simulink subsystem "PvtSubSys_HMI"  (R2020b)
settings: Solver=VariableStepAuto  StartTime=0.0  StopTime=10.0  RelTol=1e-3
undefined symbols (not defined in the file): P_HMI_LDW_LKAWarnTime, P_HMI_ObjectTypeFilter, P_HMI_WarnFormLDWReq
libraries: simulink x212, TrueDurationTime x6
(part 2 of 8)

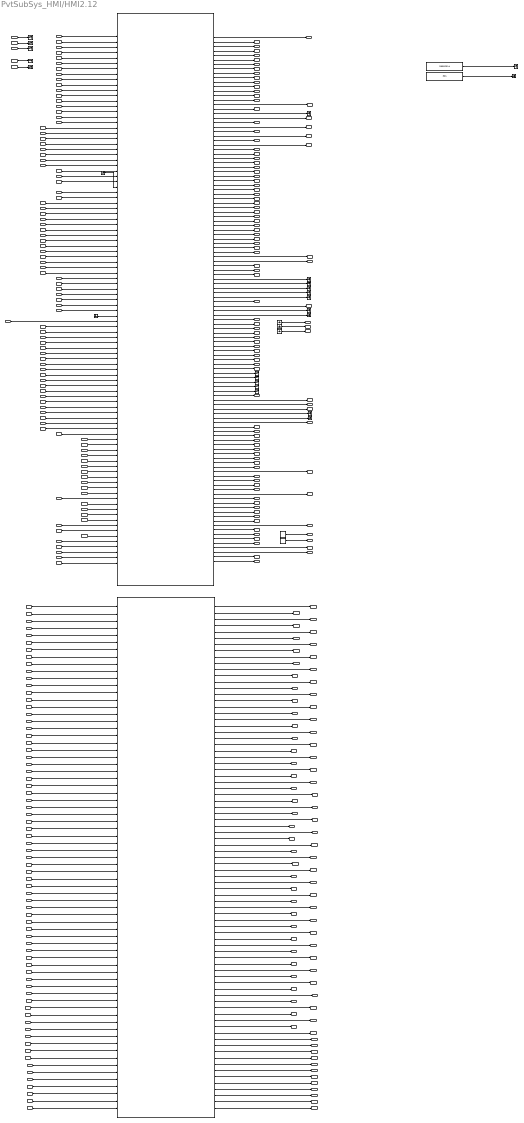
== system PvtSubSys_HMI/HMI2.12 ==
  note: 新加
  note: 与下 名字不一致
  note: 输出信号：拉出皆为输入与输出名字相同导致
      | 绿色：ACC_FD1
      | 黄色：ACC_FD2
  note: notuse
  ACCSts : Inport
  ACC_SpdSetValue : Inport  Port=2
  ACC_TimeGapSet : Inport  Port=3
  ACC_DrvOffReq : Inport  Port=4
  vSetBelowMin : Inport  Port=5
  HWAAccControlSts : Inport  Port=6
  TJASts : Inport  Port=7
  HWASts : Inport  Port=8
  HWAActive : Inport  Port=9
  ACC_HazActv : Inport  Port=10
  ACC_ModeDisp : Inport  Port=11
  ACC_ParkShiftReq : Inport  Port=12
  TJA_ModeDisp : Inport  Port=13
  HWA_ModeDisp : Inport  Port=14
  HWASlowRetreat_b : Inport  Port=15
  CruiseChauffeur_ModeDisp : Inport  Port=16
  ACCTextDisp : Inport  Port=17
  TJATextDisp : Inport  Port=18
  CCTextDisp : Inport  Port=19
  HWATextDisp : Inport  Port=20
  LCKSts : Inport  Port=21
  HandsOffWarningLevel : Inport  Port=22
  LDWState : Inport  Port=23
  LKAState : Inport  Port=24
  LKAWarning : Inport  Port=25
  ELKSts : Inport  Port=26
  LCKIESts : Inport  Port=27
  ACC_ISLResp : Inport  Port=28
  ISL_InterSysInfoDisp : Inport  Port=29
  ISLActive : Inport  Port=30
  ALC_Resp : Inport  Port=31
  HWA_SnvtySet_Resp : Inport  Port=32
  HWA_Resp : Inport  Port=33
  ICA_HandsOffSwtResp : Inport  Port=34
  TJA_ACC_SelSts : Inport  Port=35
  HWA_LaneChangeReq : Inport  Port=36
  HWA_Warning : Inport  Port=37
  HandsoffDetd : Inport  Port=38
  LSS_WarnFormSwtResp : Inport  Port=39
  DriverInloop_Monitor : Inport  Port=40
  ACC_SOS_Req : Inport  Port=41
  LaneAvailability : Inport  Port=42
  TJA_FollowSts : Inport  Port=43
  ESSSts : Inport  Port=44
  AESSts : Inport  Port=45
  HWA_TurnLightReq : Inport  Port=46
  ACC_DrvrOffDisp : Inport  Port=47
  LSSSwtReq : Inport  Port=48
  ESS_PedSwtReq : Inport  Port=49
  ESS_VehSwtReq : Inport  Port=50
  AESSwtReq : Inport  Port=51
  IFC_SnvtySet : Inport  Port=52
  ADAS_Posn_CurLane : Inport  Port=53
  NavSpdLimValue : Inport  Port=54
  NavSpdLimUnit_HUT : Inport  Port=55
  IFC_CalibrationSts : Inport  Port=56
  Camera_BlockageSts : Inport  Port=57
  ACC_Decel_Req : Inport  Port=58
  IDP0 : Inport  Port=59
  dxP0 : Inport  Port=60
  vxRelP0 : Inport  Port=61
  ACCTgtObjVy : Inport  Port=62
  axAbsGroundP0 : Inport  Port=63
  targetExistP0 : Inport  Port=64
  fu_typeP0 : Inport  Port=65
  ObjMovingStateP0 : Inport  Port=66
  Object_Orientation : Inport  Port=67
  ObjTypeP0 : Inport  Port=68
  ObjDYP0 : Inport  Port=69
  ACCTgtObjObstcl : Inport  Port=70
  ACCTgtObjAy : Inport  Port=71
  ACCTgtObjCntAlive : Inport  Port=72
  ACCTgtObjExist : Inport  Port=73
  P0HeadingAngle : Inport  Port=74
  <IDP1> : Inport  Port=75
  dxP1 : Inport  Port=76
  targetExistP1 : Inport  Port=77
  fu_typeP1 : Inport  Port=78
  ObjTypeP1 : Inport  Port=79
  ObjDYP1 : Inport  Port=80
  P1HeadingAngle : Inport  Port=81
  IDP2 : Inport  Port=82
  dxP2 : Inport  Port=83
  targetExistP2 : Inport  Port=84
  fu_typeP2 : Inport  Port=85
  ObjTypeP2 : Inport  Port=86
  ObjDYP2 : Inport  Port=87
  P2HeadingAngle : Inport  Port=88
  IDP3 : Inport  Port=89
  dxP3 : Inport  Port=90
  targetExistP3 : Inport  Port=91
  fu_typeP3 : Inport  Port=92
  ObjTypeP3 : Inport  Port=93
  ObjDYP3 : Inport  Port=94
  P3HeadingAngle : Inport  Port=95
  dyP4 : Inport  Port=96
  dxP4 : Inport  Port=97
  ObjTypeP4 : Inport  Port=98
  targetExistP4 : Inport  Port=99
  dyP5 : Inport  Port=100
  dxP5 : Inport  Port=101
  ObjTypeP5 : Inport  Port=102
  targetExistP5 : Inport  Port=103
  "L1blsLineExist " : Inport  Port=104
  L1dC0V : Inport  Port=105
  L1dC1V : Inport  Port=106
  L1dC2V : Inport  Port=107
  L1dC3V : Inport  Port=108
  L1enLineType : Inport  Port=109
  L1dDisStart : Inport  Port=110
  L1dDisFront : Inport  Port=111
  "R1blsLineExist " : Inport  Port=112
  R1dC0V : Inport  Port=113
  R1dC1V : Inport  Port=114
  R1dC2V : Inport  Port=115
  R1dC3V : Inport  Port=116
  R1enLineType : Inport  Port=117
  R1dDisStart : Inport  Port=118
  R1dDisFront : Inport  Port=119
  L2dC0V : Inport  Port=120
  L2dC1V : Inport  Port=121
  L2dC2V : Inport  Port=122
  L2dC3V : Inport  Port=123
  L2enLineType : Inport  Port=124
  L2dDisStart : Inport  Port=125
  L2dDisFront : Inport  Port=126
  L2LineExist : Inport  Port=127
  R2dC0V : Inport  Port=128
  R2dC1V : Inport  Port=129
  R2dC2V : Inport  Port=130
  R2dC3V : Inport  Port=131
  R2enLineType : Inport  Port=132
  R2dDisStart : Inport  Port=133
  R2dDisFront : Inport  Port=134
  R2LineExist : Inport  Port=135
  F_LBblsLineExist : Inport  Port=136
  F_LBdC0V : Inport  Port=137
  F_LBdC1V : Inport  Port=138
  F_LBdC2V : Inport  Port=139
  F_LBdC3V : Inport  Port=140
  F_LBenLineType : Inport  Port=141
  E1dDisStart : Inport  Port=142
  E1dDisFront : Inport  Port=143
  F_RBblsLineExist : Inport  Port=144
  F_RBdC0V : Inport  Port=145
  F_RBdC1V : Inport  Port=146
  F_RBdC2V : Inport  Port=147
  F_RBdC3V : Inport  Port=148
  F_RBenLineType : Inport  Port=149
  E2dDisFront : Inport  Port=150
  E2dDisStart : Inport  Port=151
  TunnelDistance : Inport  Port=152
  BridgeDistance : Inport  Port=153
  RampDistance : Inport  Port=154
  DrivingOnHighWay : Inport  Port=155
  RoadCurvatureFarDistance : Inport  Port=156
  RoadCurvature : Inport  Port=157
  RoadCurvatureFar : Inport  Port=158
  "Inter_AEB_TgtDecel_Req " : Inport  Port=159
  Inter_FCW_Warn : Inport  Port=160
  TSR_Sign_Long_Distance : Inport  Port=161
  DrvrState : Inport  Port=162
  MapDataValid : Inport  Port=163
  IFCHUTInterface : Inport  Port=164
  Long_ACCTakeoverReq : Inport  Port=165
  ACC_TgtObjBarDisp : Inport  Port=166
  ACC_LeTgtObjBarDisp : Inport  Port=167
  ACC_RiTgtObjBarDisp : Inport  Port=168
  LKASwtReq : Inport  Port=169
  LCKSwtReq : Inport  Port=170
  IntelligentCurveActive : Inport  Port=171
  standstill : Inport  Port=172
  Constant : Constant  Value=false
  Constant2 : Constant  Value=0  OutDataTypeStr=uint8
  Constant7 : Constant  Value=39092014  OutDataTypeStr=uint32
  Constant8 : Constant  Value=301  OutDataTypeStr=uint16
  Ground{3,10,12..14} (5 alike) : Ground
  HWA/ACC/TJA_Signal1 : Subsystem
  IFC_Signal1 : Subsystem
  TJASts1 : InportShadow  Port=7
  Terminator{1..3,5..6,9..22,24..26} (22 alike) : Terminator
  ACC_ModDisp : Outport
  TJA_ICA_ModDisp : Outport  Port=2
  HWA_ModDisp : Outport  Port=3
  ACC_InterSysInfoDisp : Outport  Port=4
  TJA_ICA_InterSysInfoDisp : Outport  Port=5
  HWA_InterSysInfoDisp : Outport  Port=6
  CruCha_ModDisp : Outport  Port=7
  CruChar_InterSysInfoDisp : Outport  Port=8
  ALCResp : Outport  Port=9
  HWAResp : Outport  Port=10
  ISL_Resp : Outport  Port=11
  ICA_HandsOffResp : Outport  Port=12
  HWAwarning : Outport  Port=13
  ACCTimeGapSet : Outport  Port=14
  ACCSpdSetValue : Outport  Port=15
  TJA_ACCSelSts : Outport  Port=16
  ACC_TakeOverReq : Outport  Port=17
  ACC_FctSts : Outport  Port=18
  ACC_EgoStatus : Outport  Port=19
  Longctrl_HazActv : Outport  Port=20
  ADAS_DriverInloop_Monitor : Outport  Port=21
  HWASnvtySetResp : Outport  Port=22
  HWA_Lane_ChangeReq : Outport  Port=23
  HWA_LaneChange : Outport  Port=24
  ACC_ObjDetecte : Outport  Port=25
  ACC_RlvTgtDetn : Outport  Port=26
  ACC_PotentialTgtDetn : Outport  Port=27
  ACC_PotentialTgtTyp : Outport  Port=28
  ACC_PotentialTgtDx : Outport  Port=29
  ACC_PotentialTgtDy : Outport  Port=30
  ACC_LeTargrtDection : Outport  Port=31
  ACC_LeTgtTyp : Outport  Port=32
  ACC_LeTgtDx : Outport  Port=33
  ACC_LeTgtDy : Outport  Port=34
  ACC_RiTargrtDetn : Outport  Port=35
  ACC_RiTgtTyp : Outport  Port=36
  ACC_RiTgtDx : Outport  Port=37
  ACC_RiTgtDy : Outport  Port=38
  ISLInterSysInfoDisp : Outport  Port=39
  Longctrl_DrvOFF_Req_DVR : Outport  Port=40
  Longctrl_ModSts_DVR : Outport  Port=41
  Longctrl_ParkShiftReq_DVR : Outport  Port=42
  ACC_RlvTgtTyp : Outport  Port=43
  ACC_RlvTgtDx : Outport  Port=44
  ACC_RlvTgtDy : Outport  Port=45
  Longctrl_HCUTrqReq_DVR : Outport  Port=46
  ALC_InterSysInfoDisp : Outport  Port=47
  Request_driveoff : Outport  Port=48
  Longctrl_VehHldReq_DVR : Outport  Port=49
  Longctrl_HCUTrqReqActive_DVR : Outport  Port=50
  IntelligentCurveAct : Outport  Port=51
  ACC_RlvTgtfusion : Outport  Port=52
  ACC_RlvTgtHeading : Outport  Port=53
  ACC_LeTgtfusion : Outport  Port=54
  ACC_LeTgtHeading : Outport  Port=55
  ACC_RiTgtfusion : Outport  Port=56
  ACC_RiTgtHeading : Outport  Port=57
  ACC_PotentialTgtfusion : Outport  Port=58
  ACC_PotentialTgtHeading : Outport  Port=59
  ACC_LeTgt_02_Dy : Outport  Port=60
  ACC_LeTgt_02_Dx : Outport  Port=61
  ACC_LeTgt_02_Typ : Outport  Port=62
  ACC_LeTargrt_02_Detn : Outport  Port=63
  ACC_RiTargrt_02_Detn : Outport  Port=64
  ACC_RiTgt_02_Dy : Outport  Port=65
  ACC_RiTgt_02_Dx : Outport  Port=66
  ACC_RiTgt_02_Typ : Outport  Port=67
  ACCTgtObjBarDisp : Outport  Port=68
  ACCLeTgtObjBarDisp : Outport  Port=69
  ACCRiTgtObjBarDisp : Outport  Port=70
  Longctrl_DrvOFF_Req : Outport  Port=71
  Longctrl_ModSts : Outport  Port=72
  Longctrl_ParkShiftReq : Outport  Port=73
  ActualTargetSpeed : Outport  Port=74
  Longctrl_VehHldReq : Outport  Port=75
  ACC_CRInterface : Outport  Port=76
  Longctrl_FuelCutOffPrevn : Outport  Port=77
  ACCTgtObjDx : Outport  Port=78
  ACCTgtObjDy : Outport  Port=79
  ACC_TgtObjObstcl : Outport  Port=80
  ACC_TgtObjExist : Outport  Port=81
  ACC_TgtObjVy : Outport  Port=82
  ACCTgtObjVx : Outport  Port=83
  ACCTgtObjAx : Outport  Port=84
  ACC_TgtObjAy : Outport  Port=85
  ACCTgtObjState : Outport  Port=86
  ACCTgtObjVideoCfmd : Outport  Port=87
  ACC_TgtObjCntAlive : Outport  Port=88
  Handsoff_Detd : Outport  Port=89
  DrvgOnHiWay : Outport  Port=90
  RoadCrvt : Outport  Port=91
  SpdLimitDst : Outport  Port=92
  RoadCrvtFar : Outport  Port=93
  RampDst : Outport  Port=94  OutDataTypeStr=uint16
  SpdLimit : Outport  Port=95
  CurveDst : Outport  Port=96
  NavSpdLimUnit : Outport  Port=97
  TunnelDst : Outport  Port=98  OutDataTypeStr=uint16
  Drvg_OnRiLane : Outport  Port=99
  BrdgDst : Outport  Port=100  OutDataTypeStr=uint16
  ACC_SOSReq : Outport  Port=101
  Map_DataValid : Outport  Port=102
  DrvrSts : Outport  Port=103
  ACCTgtObjID : Outport  Port=104
  LSSIntervention : Outport  Port=105
  LSSWarnFormResp : Outport  Port=106
  ELKResp : Outport  Port=107
  LCKResp : Outport  Port=108
  LKAResp : Outport  Port=109
  LDWResp : Outport  Port=110
  IntelligentEvaResp : Outport  Port=111
  LSSFuncSts : Outport  Port=112
  LSSErrSts : Outport  Port=113
  LSSResp : Outport  Port=114
  ELKMainState : Outport  Port=115
  LDW_LKAWarn : Outport  Port=116
  ESS_PedResp : Outport  Port=117
  ESS_VehResp : Outport  Port=118
  AESResp : Outport  Port=119
  IFC_LaneAvailability : Outport  Port=120
  LDW_LKA_Snvty : Outport  Port=121
  IFCCalibrationSts : Outport  Port=122
  IFC_HUTInterface : Outport  Port=123
  CameraBlockageSts : Outport  Port=124
  TJAFollowSts : Outport  Port=125
  IFC_LeLaneTyp : Outport  Port=126
  IFC_RiLaneTyp : Outport  Port=127
  IFC_NextLeLaneTyp : Outport  Port=128
  IFC_NextRiLaneTyp : Outport  Port=129
  IFC_LaneCurve : Outport  Port=130
  IFC_LeLane_dy : Outport  Port=131
  IFC_RiLane_dy : Outport  Port=132
  IFC_NextLeLane_dy : Outport  Port=133
  IFC_NextRiLane_dy : Outport  Port=134
  AESintervention : Outport  Port=135
  ESSintervention : Outport  Port=136
  ELKActSts : Outport  Port=137
  IntelligentEvaActSts : Outport  Port=138
  IFC_Handsoffwarn : Outport  Port=139
  AES_Sts : Outport  Port=140
  ESS_Sts : Outport  Port=141
  IFC_Line01_Dy : Outport  Port=142
  IFC_Line01_Curv : Outport  Port=143
  IFC_Line01_CurvChange : Outport  Port=144
  IFC_Line01_Type : Outport  Port=145
  IFC_Line02_Dy : Outport  Port=146
  IFC_Line02_Curv : Outport  Port=147
  IFC_Line02_CurvChange : Outport  Port=148
  IFC_Line02_Type : Outport  Port=149
  IFC_Line03_Dy : Outport  Port=150
  IFC_Line03_Curv : Outport  Port=151
  IFC_Line03_CurvChange : Outport  Port=152
  IFC_Line03_Type : Outport  Port=153
  IFC_Line04_Dy : Outport  Port=154
  IFC_Line04_Curv : Outport  Port=155
  IFC_Line04_CurvChange : Outport  Port=156
  IFC_Line04_Type : Outport  Port=157
  IFC_Roadedge01_Dy : Outport  Port=158
  IFC_Roadedge01_Curv : Outport  Port=159
  IFC_Roadedge01_CurvChange : Outport  Port=160
  IFC_Roadedge01_Type : Outport  Port=161
  IFC_Roadedge02_Dy : Outport  Port=162
  IFC_Roadedge02_Curv : Outport  Port=163
  IFC_Roadedge02_CurvChange : Outport  Port=164
  IFC_Roadedge02_Type : Outport  Port=165
  IFC_Line01_HeadingAngle : Outport  Port=166
  IFC_Line02_HeadingAngle : Outport  Port=167
  IFC_Line03_HeadingAngle : Outport  Port=168
  IFC_Line04_HeadingAngle : Outport  Port=169
  IFC_Roadedge01_HeadingAngle : Outport  Port=170
  IFC_Roadedge02_HeadingAngle : Outport  Port=171
  IFC_Line01_DxStart : Outport  Port=172
  IFC_Line01_DxEnd : Outport  Port=173
  IFC_Line02_DxStart : Outport  Port=174
  IFC_Line02_DxEnd : Outport  Port=175
  IFC_Line03_DxStart : Outport  Port=176
  IFC_Line03_DxEnd : Outport  Port=177
  IFC_Line04_DxStart : Outport  Port=178
  IFC_Line04_DxEnd : Outport  Port=179
  IFC_Roadedge01_DxStart : Outport  Port=180
  IFC_Roadedge01_DxEnd : Outport  Port=181
  IFC_Roadedge02_DxStart : Outport  Port=182
  IFC_Roadedge02_DxEnd : Outport  Port=183
  IFCVibrationWarning : Outport  Port=184
  AESErrSts : Outport  Port=185
  ESSErrSts : Outport  Port=186
  IDC_L2_EmgyLightReq : Outport  Port=187
  IDC_L2_TurnLightReq : Outport  Port=188
  IDC_L2_FWiperReq : Outport  Port=189
  wires:
  standstill/1 -> IFC_Signal1/71(standstill)
  Constant7/1 -> Terminator24/1  "HMI_SubModel_VERSION"
  Constant8/1 -> Terminator26/1  "HMI_SubModel_Number"
  ACC_DrvrOffDisp/1 -> HWA/ACC/TJA_Signal1/99(ACC_DrvrOffDisp)
  R2LineExist/1 -> IFC_Signal1/70(R2LineExist)
  L2LineExist/1 -> IFC_Signal1/69(L2LineExist)
  E2dDisFront/1 -> IFC_Signal1/68(E2dDisStart)
  E2dDisStart/1 -> IFC_Signal1/67(E2dDisFront)
  L2dDisStart/1 -> IFC_Signal1/61(L2dDisStart)
  R1dDisFront/1 -> IFC_Signal1/60(R1dDisFront)
  R1dDisStart/1 -> IFC_Signal1/59(R1dDisStart)
  L2dDisFront/1 -> IFC_Signal1/62(L2dDisFront)
  E1dDisFront/1 -> IFC_Signal1/66(E1dDisFront)
  R2dDisFront/1 -> IFC_Signal1/64(R2dDisFront)
  L1dDisFront/1 -> IFC_Signal1/58(L1dDisFront)
  L1dDisStart/1 -> IFC_Signal1/57(L1dDisStart)
  E1dDisStart/1 -> IFC_Signal1/65(E1dDisStart)
  R2dDisStart/1 -> IFC_Signal1/63(R2dDisStart)
  IFC_Signal1/81(IFC_Roadedge02_DxEnd) -> IFC_Roadedge02_DxEnd/1
  IFC_Signal1/80(IFC_Roadedge02_DxStart) -> IFC_Roadedge02_DxStart/1
  IFC_Signal1/79(IFC_Roadedge01_DxEnd) -> IFC_Roadedge01_DxEnd/1
  IFC_Signal1/78(IFC_Roadedge01_DxStart) -> IFC_Roadedge01_DxStart/1
  IFC_Signal1/77(IFC_Line04_DxEnd) -> IFC_Line04_DxEnd/1
  IFC_Signal1/76(IFC_Line04_DxStart) -> IFC_Line04_DxStart/1
  IFC_Signal1/75(IFC_Line03_DxEnd) -> IFC_Line03_DxEnd/1
  IFC_Signal1/74(IFC_Line03_DxStart) -> IFC_Line03_DxStart/1
  IFC_Signal1/73(IFC_Line02_DxEnd) -> IFC_Line02_DxEnd/1
  IFC_Signal1/72(IFC_Line02_DxStart) -> IFC_Line02_DxStart/1
  IFC_Signal1/71(IFC_Line01_DxEnd) -> IFC_Line01_DxEnd/1
  IFC_Signal1/70(IFC_Line01_DxStart) -> IFC_Line01_DxStart/1
  HWA_TurnLightReq/1 -> HWA/ACC/TJA_Signal1/98(HWA_TurnLightReq)
  ACC_RiTgtObjBarDisp/1 -> HWA/ACC/TJA_Signal1/97(ACC_RiTgtObjBarDisp1)
  ACC_LeTgtObjBarDisp/1 -> HWA/ACC/TJA_Signal1/96(ACC_LeTgtObjBarDisp1)
  ACC_TgtObjBarDisp/1 -> HWA/ACC/TJA_Signal1/95(ACC_TgtObjBarDisp1)
  Constant2/1 -> IDC_L2_FWiperReq/1  "IDC_L2_FWiperReq"
  HWA/ACC/TJA_Signal1/118(HWA_TurnLightReqout) -> IDC_L2_TurnLightReq/1  "IDC_L2_TurnLightReq"
  Constant/1 -> IDC_L2_EmgyLightReq/1  "IDC_L2_EmgyLightReq"
  LCKSwtReq/1 -> IFC_Signal1/56(LCKSwtReq)
  LKASwtReq/1 -> IFC_Signal1/55(LKASwtReq)
  F_LBblsLineExist/1 -> IFC_Signal1/43(F_LBblsLineExist)
  F_RBblsLineExist/1 -> IFC_Signal1/49(F_RBblsLineExist)
  LSSSwtReq/1 -> IFC_Signal1/1(LSSSwtReq)
  "R1blsLineExist "/1 -> IFC_Signal1/29("R1blsLineExist ")
  "L1blsLineExist "/1 -> IFC_Signal1/27("L1blsLineExist ")
  HandsOffWarningLevel/1 -> HWA/ACC/TJA_Signal1/94(HandsOffWarningLevel)
  HWA/ACC/TJA_Signal1/4(HWA_InterSysInfoDisp) -> HWA_InterSysInfoDisp/1  "HWA_InterSysInfoDisp"
  HWATextDisp/1 -> HWA/ACC/TJA_Signal1/93(HWATextDisp)
  Ground14/1 -> Longctrl_HCUTrqReq_DVR/1  "Longctrl_HCUTrqReq_DVR"
  Ground13/1 -> IntelligentCurveAct/1  "IntelligentCurveAct"
  Ground12/1 -> Longctrl_HCUTrqReqActive_DVR/1  "Longctrl_HCUTrqReqActive_DVR"
  ACC_Decel_Req/1 -> HWA/ACC/TJA_Signal1/51(ACC_Decel_ReqValue)
  HWA/ACC/TJA_Signal1/86(Longctrl_HCUTrqReq) -> Terminator22/1
  HWA/ACC/TJA_Signal1/85(Longctrl_HCUTrqReqActive) -> Terminator21/1
  HWA/ACC/TJA_Signal1/80(Longctrl_Decel_ReqValue) -> Terminator20/1
  HWA/ACC/TJA_Signal1/79(Longctrl_DecelToStopReq) -> Terminator19/1
  HWA/ACC/TJA_Signal1/78(Longctrl_EngTrqReqActive) -> Terminator18/1
  HWA/ACC/TJA_Signal1/77(Longctrl_EngTrqReq) -> Terminator17/1
  HWA/ACC/TJA_Signal1/76(Longctrl_Decel_Req) -> Terminator16/1
  HWA/ACC/TJA_Signal1/63(Longctrl_HCUTrqReq_DVR) -> Terminator15/1  "Longctrl_HCUTrqReq_DVR"
  HWA/ACC/TJA_Signal1/62(Longctrl_HCUTrqReqActive_DVR) -> Terminator14/1  "Longctrl_HCUTrqReqActive_DVR"
  HWA/ACC/TJA_Signal1/59(Longctrl_Decel_ReqValue_DVR) -> Terminator13/1  "Longctrl_Decel_ReqValue_DVR"
  HWA/ACC/TJA_Signal1/58(Longctrl_DecelToStopReq_DVR) -> Terminator12/1  "Longctrl_DecelToStopReq_DVR"
  HWA/ACC/TJA_Signal1/57(Longctrl_EngTrqReqActive_DVR) -> Terminator11/1  "Longctrl_EngTrqReqActive_DVR"
  HWA/ACC/TJA_Signal1/56(Longctrl_EngTrqReq_DVR) -> Terminator6/1  "Longctrl_EngTrqReq_DVR"
  HWA/ACC/TJA_Signal1/55(Longctrl_Decel_Req_DVR) -> Terminator5/1  "Longctrl_Decel_Req_DVR"
  HWA/ACC/TJA_Signal1/51(ACCRiTgtObjBarDisp) -> ACCRiTgtObjBarDisp/1  "ACCRiTgtObjBarDisp"
  HWA/ACC/TJA_Signal1/50(ACCLeTgtObjBarDisp) -> ACCLeTgtObjBarDisp/1  "ACCLeTgtObjBarDisp"
  CCTextDisp/1 -> HWA/ACC/TJA_Signal1/54(CCTextDisp)
  Ground10/1 -> HWA/ACC/TJA_Signal1/53(HCUTrqReqActive)
  IDP3/1 -> HWA/ACC/TJA_Signal1/50(IDP3)
  <IDP1>/1 -> HWA/ACC/TJA_Signal1/49(IDP1)
  IDP2/1 -> HWA/ACC/TJA_Signal1/48(IDP2)
  Ground3/1 -> HWA/ACC/TJA_Signal1/29(ACC_Decel_Req)
  IntelligentCurveActive/1 -> HWA/ACC/TJA_Signal1/17(IntelligentCurveActive)
  Long_ACCTakeoverReq/1 -> HWA/ACC/TJA_Signal1/15(ACC_TakeOverReq)
  IFC_Signal1/24(ESSErrSts) -> ESSErrSts/1  "ESSErrSts"
  IFC_Signal1/23(ESS_Sts) -> ESS_Sts/1  "ESSSts"
  IFC_Signal1/21(AESErrSts) -> AESErrSts/1
  IFC_Signal1/20(AES_Sts) -> AES_Sts/1  "AESSts"
  AESSts/1 -> IFC_Signal1/12(AESSts)
  HWA/ACC/TJA_Signal1/117(IFC_Handsoffwarn) -> IFC_Handsoffwarn/1  "IFC_Handsoffwarn"
  F_RBenLineType/1 -> IFC_Signal1/54(F_RBenLineType)
  F_RBdC3V/1 -> IFC_Signal1/53(F_RBdC3V)
  F_RBdC2V/1 -> IFC_Signal1/52(F_RBdC2V)
  F_RBdC1V/1 -> IFC_Signal1/51(F_RBdC1V)
  F_RBdC0V/1 -> IFC_Signal1/50(F_RBdC0V)
  F_LBenLineType/1 -> IFC_Signal1/48(F_LBenLineType)
  F_LBdC3V/1 -> IFC_Signal1/47(F_LBdC3V)
  F_LBdC2V/1 -> IFC_Signal1/46(F_LBdC2V)
  F_LBdC1V/1 -> IFC_Signal1/45(F_LBdC1V)
  F_LBdC0V/1 -> IFC_Signal1/44(F_LBdC0V)
  R2dC1V/1 -> IFC_Signal1/42(R2dC1V)
  R2dC3V/1 -> IFC_Signal1/41(R2dC3V)
  R2dC2V/1 -> IFC_Signal1/40(R2dC2V)
  L2dC1V/1 -> IFC_Signal1/39(L2dC1V)
  L2dC3V/1 -> IFC_Signal1/38(L2dC3V)
  L2dC2V/1 -> IFC_Signal1/37(L2dC2V)
  R1dC1V/1 -> IFC_Signal1/36(R1dC1V)
  R1dC3V/1 -> IFC_Signal1/35(R1dC3V)
  L1dC1V/1 -> IFC_Signal1/34(L1dC1V)
  L1dC3V/1 -> IFC_Signal1/33(L1dC3V)
  IFC_Signal1/69(IFC_Roadedge02_Type) -> IFC_Roadedge02_Type/1  "IFC_Roadedge02_Type"
  IFC_Signal1/68(IFC_Roadedge02_CurvChange) -> IFC_Roadedge02_CurvChange/1  "IFC_Roadedge02_CurvChange"
  IFC_Signal1/67(IFC_Roadedge02_Curv) -> IFC_Roadedge02_Curv/1  "IFC_Roadedge02_Curv"
  IFC_Signal1/66(IFC_Roadedge02_HeadingAngle) -> IFC_Roadedge02_HeadingAngle/1  "IFC_Roadedge02_HeadingAngle"
  IFC_Signal1/65(IFC_Roadedge02_Dy) -> IFC_Roadedge02_Dy/1  "IFC_Roadedge02_Dy"
  IFC_Signal1/64(IFC_Roadedge01_Type) -> IFC_Roadedge01_Type/1  "IFC_Roadedge01_Type"
  IFC_Signal1/63(IFC_Roadedge01_CurvChange) -> IFC_Roadedge01_CurvChange/1  "IFC_Roadedge01_CurvChange"
  IFC_Signal1/62(IFC_Roadedge01_Curv) -> IFC_Roadedge01_Curv/1  "IFC_Roadedge01_Curv"
  IFC_Signal1/61(IFC_Roadedge01_HeadingAngle) -> IFC_Roadedge01_HeadingAngle/1  "IFC_Roadedge01_HeadingAngle"
  IFC_Signal1/60(IFC_Roadedge01_Dy) -> IFC_Roadedge01_Dy/1  "IFC_Roadedge01_Dy"
  IFC_Signal1/59(IFC_Line04_HeadingAngle) -> IFC_Line04_HeadingAngle/1  "IFC_Line04_HeadingAngle"
  IFC_Signal1/58(IFC_Line04_CurvChange) -> IFC_Line04_CurvChange/1  "IFC_Line04_CurvChange"
  IFC_Signal1/57(IFC_Line04_Curv) -> IFC_Line04_Curv/1  "IFC_Line04_Curv"
  IFC_Signal1/56(IFC_Line03_HeadingAngle) -> IFC_Line03_HeadingAngle/1  "IFC_Line03_HeadingAngle"
  IFC_Signal1/55(IFC_Line03_CurvChange) -> IFC_Line03_CurvChange/1  "IFC_Line03_CurvChange"
  IFC_Signal1/54(IFC_Line03_Curv) -> IFC_Line03_Curv/1  "IFC_Line03_Curv"
  IFC_Signal1/53(IFC_Line02_HeadingAngle) -> IFC_Line02_HeadingAngle/1  "IFC_Line02_HeadingAngle"
  IFC_Signal1/52(IFC_Line02_CurvChange) -> IFC_Line02_CurvChange/1  "IFC_Line02_CurvChange"
  IFC_Signal1/51(IFC_Line01_HeadingAngle) -> IFC_Line01_HeadingAngle/1  "IFC_Line01_HeadingAngle"
  IFC_Signal1/50(IFC_Line01_CurvChange) -> IFC_Line01_CurvChange/1  "IFC_Line01_CurvChange"
  IFC_Signal1/49(IFC_Line04_Dy) -> IFC_Line04_Dy/1  "IFC_Line04_Dy"
  IFC_Signal1/47(IFC_Line03_Dy) -> IFC_Line03_Dy/1  "IFC_Line03_Dy"
  IFC_Signal1/45(IFC_Line02_Dy) -> IFC_Line02_Dy/1  "IFC_Line02_Dy"
  IFC_Signal1/43(IFC_Line01_Dy) -> IFC_Line01_Dy/1  "IFC_Line01_Dy"
  IFC_Signal1/41(IFC_Line02_Curv) -> IFC_Line02_Curv/1  "IFC_Line02_Curv"
  IFC_Signal1/39(IFC_Line01_Curv) -> IFC_Line01_Curv/1  "IFC_Line01_Curv"
  IFC_Signal1/38(IFC_Line04_Type) -> IFC_Line04_Type/1  "IFC_Line04_Type"
  IFC_Signal1/36(IFC_Line03_Type) -> IFC_Line03_Type/1  "IFC_Line03_Type"
  IFC_Signal1/34(IFC_Line02_Type) -> IFC_Line02_Type/1  "IFC_Line02_Type"
  IFC_Signal1/32(IFC_Line01_Type) -> IFC_Line01_Type/1  "IFC_Line01_Type"
  HWA/ACC/TJA_Signal1/71(ACC_RiTargrt_02_Detn) -> ACC_RiTargrt_02_Detn/1  "ACC_RiTargrt_02_Detn"
  HWA/ACC/TJA_Signal1/70(ACC_RiTgt_02_Typ) -> ACC_RiTgt_02_Typ/1  "ACC_RiTgt_02_Typ"
  HWA/ACC/TJA_Signal1/69(ACC_RiTgt_02_Dx) -> ACC_RiTgt_02_Dx/1  "ACC_RiTgt_02_Dx"
  HWA/ACC/TJA_Signal1/68(ACC_RiTgt_02_Dy) -> ACC_RiTgt_02_Dy/1  "ACC_RiTgt_02_Dy"
  HWA/ACC/TJA_Signal1/67(ACC_LeTargrt_02_Detn) -> ACC_LeTargrt_02_Detn/1  "ACC_LeTargrt_02_Detn"
  HWA/ACC/TJA_Signal1/66(ACC_LeTgt_02_Typ) -> ACC_LeTgt_02_Typ/1  "ACC_LeTgt_02_Typ"
  HWA/ACC/TJA_Signal1/65(ACC_LeTgt_02_Dx) -> ACC_LeTgt_02_Dx/1  "ACC_LeTgt_02_Dx"
  HWA/ACC/TJA_Signal1/64(ACC_LeTgt_02_Dy) -> ACC_LeTgt_02_Dy/1  "ACC_LeTgt_02_Dy"
  targetExistP5/1 -> HWA/ACC/TJA_Signal1/62(targetExistP5)
  ObjTypeP5/1 -> HWA/ACC/TJA_Signal1/61(ObjTypeP5)
  dxP5/1 -> HWA/ACC/TJA_Signal1/60(dxP5)
  dyP5/1 -> HWA/ACC/TJA_Signal1/59(dyP5)
  targetExistP4/1 -> HWA/ACC/TJA_Signal1/58(targetExistP4)
  ObjTypeP4/1 -> HWA/ACC/TJA_Signal1/57(ObjTypeP4)
  dxP4/1 -> HWA/ACC/TJA_Signal1/56(dxP4)
  dyP4/1 -> HWA/ACC/TJA_Signal1/55(dyP4)
  LKAState/1 -> IFC_Signal1/3(LKAState)
  LCKSts/1 -> IFC_Signal1/4(LCKState)
  ELKSts/1 -> IFC_Signal1/5(ELKSts)
  TJASts1/1 -> IFC_Signal1/8(TJAState)
  IFC_Signal1/25(IFC_LaneAvailability) -> IFC_LaneAvailability/1  "LaneAvailability"
  LKAWarning/1 -> IFC_Signal1/6(LKAWarning)
  HWASlowRetreat_b/1 -> Terminator9/1
  LCKIESts/1 -> IFC_Signal1/7(LCKIESts)
  LDWState/1 -> IFC_Signal1/2(LDWState)
  IFC_Signal1/46(IFC_NextLeLane_dy) -> IFC_NextLeLane_dy/1  "IFC_NextLeLane_dy"
  IFC_Signal1/35(IFC_NextLeLaneTyp) -> IFC_NextLeLaneTyp/1  "IFC_NextLeLaneTyp"
  LSS_WarnFormSwtResp/1 -> IFC_Signal1/9(LSS_WarnFormSwtReq)
  IFC_Signal1/26(LDW_LKA_Snvty) -> LDW_LKA_Snvty/1  "LDW_LKA_Snvty"
  L1enLineType/1 -> IFC_Signal1/21(L1enLineType)
  IFC_Signal1/29(Camera_BlockageSts) -> CameraBlockageSts/1  "CameraBlockageSts"
  Camera_BlockageSts/1 -> IFC_Signal1/19(CameraBlockageSts)
  ESS_VehSwtReq/1 -> IFC_Signal1/11(ESS_VehSwtReq)
  AESSwtReq/1 -> IFC_Signal1/13(AESSwtReq)
  TJA_FollowSts/1 -> IFC_Signal1/20(TJA_FollowSts)
  LaneAvailability/1 -> IFC_Signal1/15(LaneAvailability)
  IFC_Signal1/1(LSSFuncSts) -> LSSFuncSts/1  "LSSFuncSts"
  IFCHUTInterface/1 -> IFC_Signal1/18(IFCHUTInterface)
  ESS_PedSwtReq/1 -> IFC_Signal1/10(ESS_PedSwtReq)
  IFC_SnvtySet/1 -> IFC_Signal1/16(IFC_SnvtySet)
  L1dC0V/1 -> IFC_Signal1/28(L1dC0V)
  IFC_CalibrationSts/1 -> IFC_Signal1/17(IFCCalibrationSts)
  R1dC2V/1 -> IFC_Signal1/26(R1dC2V)
  R2dC0V/1 -> IFC_Signal1/32(R2dC0V)
  L1dC2V/1 -> IFC_Signal1/25(L1dC2V)
  R1dC0V/1 -> IFC_Signal1/30(R1dC0V)
  ESSSts/1 -> IFC_Signal1/14(ESSSts)
  R2enLineType/1 -> IFC_Signal1/24(R2enLineType)
  L2dC0V/1 -> IFC_Signal1/31(L2dC0V)
  R1enLineType/1 -> IFC_Signal1/22(R1enLineType)
  IFC_Signal1/14(LDW_LKAWarn) -> LDW_LKAWarn/1  "LDW_LKAWarn"
  L2enLineType/1 -> IFC_Signal1/23(L2enLineType)
  HWAAccControlSts/1 -> Terminator1/1
  vSetBelowMin/1 -> Terminator2/1
  ISLActive/1 -> Terminator3/1
  HWAActive/1 -> Terminator10/1
  IFC_Signal1/28(IFC_HUTInterface) -> IFC_HUTInterface/1  "IFCHUTInterface"
  IFC_Signal1/7(LCKResp) -> LCKResp/1  "LCKResp"
  IFC_Signal1/48(IFC_NextRiLane_dy) -> IFC_NextRiLane_dy/1  "IFC_NextRiLane_dy"
  IFC_Signal1/2(LSSErrSts) -> LSSErrSts/1  "LSSErrSts"
  IFC_Signal1/6(ELKResp) -> ELKResp/1  "ELKResp"
  IFC_Signal1/31(IFC_LeLaneTyp) -> IFC_LeLaneTyp/1  "IFC_LeLaneTyp"
  IFC_Signal1/3(LSSResp) -> LSSResp/1  "LSSResp"
  IFC_Signal1/10(IntelligentEvaResp) -> IntelligentEvaResp/1  "IntelligentEvaResp"
  IFC_Signal1/4(LSSIntervention) -> LSSIntervention/1  "LSSIntervention"
  IFC_Signal1/9(LDWResp) -> LDWResp/1  "LDWResp"
  IFC_Signal1/8(LKAResp) -> LKAResp/1  "LKAResp"
  IFC_Signal1/16(ESS_PedResp) -> ESS_PedResp/1  "ESS_PedResp"
  IFC_Signal1/12(ELKMainState) -> ELKMainState/1  "ELKMainState"
  IFC_Signal1/5(LSSWarnFormResp) -> LSSWarnFormResp/1  "LSSWarnFormResp"
  IFC_Signal1/18(AESResp) -> AESResp/1  "AESResp"
  IFC_Signal1/15(IFCVibrationWarning) -> IFCVibrationWarning/1
  IFC_Signal1/30(TJAFollowSts) -> TJAFollowSts/1  "TJA_FollowSts"
  IFC_Signal1/17(ESS_VehResp) -> ESS_VehResp/1  "ESS_VehResp"
  IFC_Signal1/27(IFC_CalibrationSts) -> IFCCalibrationSts/1  "IFCCalibrationSts"
  IFC_Signal1/42(IFC_LeLane_dy) -> IFC_LeLane_dy/1  "IFC_LeLane_dy"
  IFC_Signal1/37(IFC_NextRiLaneTyp) -> IFC_NextRiLaneTyp/1  "IFC_NextRiLaneTyp"
  IFC_Signal1/44(IFC_RiLane_dy) -> IFC_RiLane_dy/1  "IFC_RiLane_dy"
  IFC_Signal1/33(IFC_RiLaneTyp) -> IFC_RiLaneTyp/1  "IFC_RiLaneTyp"
  IFC_Signal1/19(AESintervention) -> AESintervention/1  "AESintervention"
  IFC_Signal1/40(IFC_LaneCurve) -> IFC_LaneCurve/1  "IFC_LaneCurve"
  IFC_Signal1/22(ESSintervention) -> ESSintervention/1  "ESSintervention"
  IFC_Signal1/11(IntelligentEvaActSts) -> IntelligentEvaActSts/1  "IntelligentEvaActSts"
  IFC_Signal1/13(ELKActSts) -> ELKActSts/1  "ELKActSts"
  HWA/ACC/TJA_Signal1/116(CruChar_InterSysInfoDisp) -> CruChar_InterSysInfoDisp/1  "CruChar_InterSysInfoDisp"
  HWA/ACC/TJA_Signal1/115(CruCha_ModDisp) -> CruCha_ModDisp/1  "CruCha_ModDisp"
  HWA/ACC/TJA_Signal1/114(DrvrSts) -> DrvrSts/1  "DrvrSts"
  HWA/ACC/TJA_Signal1/113(Map_DataValid) -> Map_DataValid/1  "Map_DataValid"
  HWA/ACC/TJA_Signal1/112(ACC_SOSReq) -> ACC_SOSReq/1  "ACC_SOSReq"
  HWA/ACC/TJA_Signal1/111(BrdgDst) -> BrdgDst/1  "BrdgDst"
  HWA/ACC/TJA_Signal1/110(Drvg_OnRiLane) -> Drvg_OnRiLane/1  "Drvg_OnRiLane"
  HWA/ACC/TJA_Signal1/109(TunnelDst) -> TunnelDst/1  "TunnelDst"
  HWA/ACC/TJA_Signal1/108(NavSpdLimUnit) -> NavSpdLimUnit/1  "NavSpdLimUnit"
  HWA/ACC/TJA_Signal1/107(CurveDst) -> CurveDst/1  "CurveDst"
  HWA/ACC/TJA_Signal1/106(SpdLimit) -> SpdLimit/1  "SpdLimit"
  HWA/ACC/TJA_Signal1/105(RampDst) -> RampDst/1  "RampDst"
  HWA/ACC/TJA_Signal1/104(RoadCrvtFar) -> RoadCrvtFar/1  "RoadCrvtFar"
  HWA/ACC/TJA_Signal1/103(SpdLimitDst) -> SpdLimitDst/1  "SpdLimitDst"
  HWA/ACC/TJA_Signal1/102(RoadCrvt) -> RoadCrvt/1  "RoadCrvt"
  HWA/ACC/TJA_Signal1/101(DrvgOnHiWay) -> DrvgOnHiWay/1  "DrvgOnHiWay"
  HWA/ACC/TJA_Signal1/100(Handsoff_Detd) -> Handsoff_Detd/1  "Handsoff_Detd"
  HWA/ACC/TJA_Signal1/99(ACC_TgtObjCntAlive) -> ACC_TgtObjCntAlive/1  "ACCTgtObjCntAlive"
  HWA/ACC/TJA_Signal1/98(ACCTgtObjVideoCfmd) -> ACCTgtObjVideoCfmd/1  "ACCTgtObjVideoCfmd"
  HWA/ACC/TJA_Signal1/97(ACCTgtObjState) -> ACCTgtObjState/1  "ACCTgtObjState"
  HWA/ACC/TJA_Signal1/96(ACC_TgtObjAy) -> ACC_TgtObjAy/1  "ACCTgtObjAy"
  HWA/ACC/TJA_Signal1/95(ACCTgtObjAx) -> ACCTgtObjAx/1  "ACCTgtObjAx"
  HWA/ACC/TJA_Signal1/94(ACCTgtObjVx) -> ACCTgtObjVx/1  "ACCTgtObjVx"
  HWA/ACC/TJA_Signal1/93(ACC_TgtObjVy) -> ACC_TgtObjVy/1  "ACCTgtObjVy"
  HWA/ACC/TJA_Signal1/92(ACC_TgtObjExist) -> ACC_TgtObjExist/1  "ACCTgtObjExist"
  HWA/ACC/TJA_Signal1/91(ACC_TgtObjObstcl) -> ACC_TgtObjObstcl/1  "ACCTgtObjObstcl"
  HWA/ACC/TJA_Signal1/90(ACCTgtObjDy) -> ACCTgtObjDy/1  "ACCTgtObjDy"
  HWA/ACC/TJA_Signal1/73(ACC_RlvTgtDy) -> ACC_RlvTgtDy/1  "ACC_RlvTgtDy"
  HWA/ACC/TJA_Signal1/89(ACCTgtObjDx) -> ACCTgtObjDx/1  "ACCTgtObjDx"
  HWA/ACC/TJA_Signal1/72(ACC_RlvTgtDx) -> ACC_RlvTgtDx/1  "ACC_RlvTgtDx"
  HWA/ACC/TJA_Signal1/88(ACCTgtObjID) -> ACCTgtObjID/1  "ACCTgtObjID"
  HWA/ACC/TJA_Signal1/87(Longctrl_FuelCutOffPrevn) -> Longctrl_FuelCutOffPrevn/1  "Longctrl_FuelCutOffPrevn"
  HWA/ACC/TJA_Signal1/84(ACC_CRInterface) -> ACC_CRInterface/1  "ACC_CRInterface"
  HWA/ACC/TJA_Signal1/61(Longctrl_VehHldReq_DVR) -> Longctrl_VehHldReq_DVR/1  "Longctrl_VehHldReq_DVR"
  HWA/ACC/TJA_Signal1/83(Longctrl_VehHldReq) -> Longctrl_VehHldReq/1  "Longctrl_VehHldReq"
  HWA/ACC/TJA_Signal1/82(ActualTargetSpeed) -> ActualTargetSpeed/1  "ActualTargetSpeed"
  HWA/ACC/TJA_Signal1/60(Longctrl_ParkShiftReq_DVR) -> Longctrl_ParkShiftReq_DVR/1  "Longctrl_ParkShiftReq_DVR"
  HWA/ACC/TJA_Signal1/81(Longctrl_ParkShiftReq) -> Longctrl_ParkShiftReq/1  "Longctrl_ParkShiftReq"
  HWA/ACC/TJA_Signal1/54(Longctrl_ModSts_DVR) -> Longctrl_ModSts_DVR/1  "Longctrl_ModSts_DVR"
  HWA/ACC/TJA_Signal1/75(Longctrl_ModSts) -> Longctrl_ModSts/1  "Longctrl_ModSts"
  HWA/ACC/TJA_Signal1/53(Request_driveoff) -> Request_driveoff/1  "Request_driveoff"
  HWA/ACC/TJA_Signal1/74(Longctrl_DrvOFF_Req) -> Longctrl_DrvOFF_Req/1  "Longctrl_DrvOFF_Req"
  HWA/ACC/TJA_Signal1/52(Longctrl_DrvOFF_Req_DVR) -> Longctrl_DrvOFF_Req_DVR/1  "Longctrl_DrvOFF_Req_DVR"
  HWA/ACC/TJA_Signal1/49(ISLInterSysInfoDisp) -> ISLInterSysInfoDisp/1  "ISLInterSysInfoDisp"
  HWA/ACC/TJA_Signal1/48(ACC_RiTgtDy) -> ACC_RiTgtDy/1  "ACC_RiTgtDy"
  HWA/ACC/TJA_Signal1/47(ACC_RiTgtDx) -> ACC_RiTgtDx/1  "ACC_RiTgtDx"
  HWA/ACC/TJA_Signal1/46(ACC_RiTgtTyp) -> ACC_RiTgtTyp/1  "ACC_RiTgtTyp"
  HWA/ACC/TJA_Signal1/45(ACC_RiTargrtDetn) -> ACC_RiTargrtDetn/1  "ACC_RiTargrtDetn"
  HWA/ACC/TJA_Signal1/44(ACC_LeTgtDy) -> ACC_LeTgtDy/1  "ACC_LeTgtDy"
  HWA/ACC/TJA_Signal1/43(ACC_LeTgtDx) -> ACC_LeTgtDx/1  "ACC_LeTgtDx"
  HWA/ACC/TJA_Signal1/42(ACC_LeTgtTyp) -> ACC_LeTgtTyp/1  "ACC_LeTgtTyp"
  HWA/ACC/TJA_Signal1/41(ACC_LeTargrtDection) -> ACC_LeTargrtDection/1  "ACC_LeTargrtDection"
  HWA/ACC/TJA_Signal1/40(ACC_PotentialTgtDy) -> ACC_PotentialTgtDy/1  "ACC_PotentialTgtDy"
  HWA/ACC/TJA_Signal1/39(ACC_PotentialTgtDx) -> ACC_PotentialTgtDx/1  "ACC_PotentialTgtDx"
  HWA/ACC/TJA_Signal1/38(ACC_PotentialTgtTyp) -> ACC_PotentialTgtTyp/1  "ACC_PotentialTgtTyp"
  HWA/ACC/TJA_Signal1/37(ACC_PotentialTgtDetn) -> ACC_PotentialTgtDetn/1  "ACC_PotentialTgtDetn"
  HWA/ACC/TJA_Signal1/36(ACC_RlvTgtTyp) -> ACC_RlvTgtTyp/1  "ACC_RlvTgtTyp"
  HWA/ACC/TJA_Signal1/35(ACC_RlvTgtDetn) -> ACC_RlvTgtDetn/1  "ACC_RlvTgtDetn"
  HWA/ACC/TJA_Signal1/34(ACC_ObjDetecte) -> ACC_ObjDetecte/1  "ACC_ObjDetecte"
  HWA/ACC/TJA_Signal1/33(ICA_HandsOffResp) -> ICA_HandsOffResp/1  "ICA_HandsOffResp"
  HWA/ACC/TJA_Signal1/32(ISL_Resp) -> ISL_Resp/1  "ISL_Resp"
  HWA/ACC/TJA_Signal1/31(ACC_EgoStatus) -> ACC_EgoStatus/1  "ACC_EgoStatus"
  HWA/ACC/TJA_Signal1/30(HWA_LaneChange) -> HWA_LaneChange/1  "HWA_LaneChange"
  HWA/ACC/TJA_Signal1/29(HWA_Lane_ChangeReq) -> HWA_Lane_ChangeReq/1  "HWA_Lane_ChangeReq"
  HWA/ACC/TJA_Signal1/28(HWASnvtySetResp) -> HWASnvtySetResp/1  "HWASnvtySetResp"
  HWA/ACC/TJA_Signal1/27(ADAS_DriverInloop_Monitor) -> ADAS_DriverInloop_Monitor/1  "ADAS_DriverInloop_Monitor"
  HWA/ACC/TJA_Signal1/26(ACC_PotentialTgtHeading) -> ACC_PotentialTgtHeading/1  "ACC_PotentialTgtHeading"
  HWA/ACC/TJA_Signal1/25(ACC_PotentialTgtfusion) -> ACC_PotentialTgtfusion/1  "ACC_PotentialTgtfusion"
  HWA/ACC/TJA_Signal1/24(ACC_RiTgtHeading) -> ACC_RiTgtHeading/1  "ACC_RiTgtHeading"
  HWA/ACC/TJA_Signal1/23(ACC_RiTgtfusion) -> ACC_RiTgtfusion/1  "ACC_RiTgtfusion"
  HWA/ACC/TJA_Signal1/22(ACC_LeTgtHeading) -> ACC_LeTgtHeading/1  "ACC_LeTgtHeading"
  HWA/ACC/TJA_Signal1/21(ACC_LeTgtfusion) -> ACC_LeTgtfusion/1  "ACC_LeTgtfusion"
  HWA/ACC/TJA_Signal1/20(ACC_RlvTgtHeading) -> ACC_RlvTgtHeading/1  "ACC_RlvTgtHeading"
  HWA/ACC/TJA_Signal1/19(ACC_RlvTgtfusion) -> ACC_RlvTgtfusion/1  "ACC_RlvTgtfusion"
  HWA/ACC/TJA_Signal1/18(IntelligentCurveAct) -> Terminator25/1  "IntelligentCurveAct"
  HWA/ACC/TJA_Signal1/17(Longctrl_HazActv) -> Longctrl_HazActv/1  "Longctrl_HazActv"
  HWA/ACC/TJA_Signal1/16(ACCTgtObjBarDisp) -> ACCTgtObjBarDisp/1  "ACCTgtObjBarDisp"
  HWA/ACC/TJA_Signal1/15(ACC_FctSts) -> ACC_FctSts/1  "ACC_FctSts"
  HWA/ACC/TJA_Signal1/14(ACCTakeOverReq) -> ACC_TakeOverReq/1  "ACCTakeOverReq"
  HWA/ACC/TJA_Signal1/13(TJA_ACCSelSts) -> TJA_ACCSelSts/1  "TJA_ACCSelSts"
  HWA/ACC/TJA_Signal1/12(ACCSpdSetValue) -> ACCSpdSetValue/1  "ACCSpdSetValue"
  HWA/ACC/TJA_Signal1/11(ACCTimeGapSet) -> ACCTimeGapSet/1  "ACCTimeGapSet"
  HWA/ACC/TJA_Signal1/10(HWAwarning) -> HWAwarning/1  "HWAwarning"
  HWA/ACC/TJA_Signal1/9(HWAResp) -> HWAResp/1  "HWAResp"
  HWA/ACC/TJA_Signal1/8(ALCResp) -> ALCResp/1  "ALCResp"
  HWA/ACC/TJA_Signal1/7(TJA_ICA_InterSysInfoDisp) -> TJA_ICA_InterSysInfoDisp/1  "TJA_ICA_InterSysInfoDisp"
  HWA/ACC/TJA_Signal1/6(ACC_InterSysInfoDisp) -> ACC_InterSysInfoDisp/1  "ACC_InterSysInfoDisp"
  HWA/ACC/TJA_Signal1/5(HWA_ModDisp) -> HWA_ModDisp/1  "HWA_ModDisp"
  HWA/ACC/TJA_Signal1/3(TJA_ICA_ModDisp) -> TJA_ICA_ModDisp/1  "TJA_ICA_ModDisp"
  HWA/ACC/TJA_Signal1/2(ACC_ModDisp) -> ACC_ModDisp/1  "ACC_ModDisp"
  HWA/ACC/TJA_Signal1/1(ALC_InterSysInfoDisp) -> ALC_InterSysInfoDisp/1  "ALC_InterSysInfoDisp"
  CruiseChauffeur_ModeDisp/1 -> HWA/ACC/TJA_Signal1/92(CruiseChauffeur_ModeDisp)
  Inter_FCW_Warn/1 -> HWA/ACC/TJA_Signal1/91(Inter_FCW_Warn)
  "Inter_AEB_TgtDecel_Req "/1 -> HWA/ACC/TJA_Signal1/90("Inter_AEB_TgtDecel_Req ")
  DrvrState/1 -> HWA/ACC/TJA_Signal1/89(DrvrState)
  MapDataValid/1 -> HWA/ACC/TJA_Signal1/88(MapDataValid)
  ACC_SOS_Req/1 -> HWA/ACC/TJA_Signal1/87(ACC_SOS_Req)
  BridgeDistance/1 -> HWA/ACC/TJA_Signal1/86(BridgeDistance)
  ADAS_Posn_CurLane/1 -> HWA/ACC/TJA_Signal1/85(ADAS_Posn_CurLane)
  TunnelDistance/1 -> HWA/ACC/TJA_Signal1/84(TunnelDistance)
  NavSpdLimUnit_HUT/1 -> HWA/ACC/TJA_Signal1/83(NavSpdLimUnit_HUT)
  RoadCurvatureFarDistance/1 -> HWA/ACC/TJA_Signal1/82(RoadCurvatureFarDistance)
  NavSpdLimValue/1 -> HWA/ACC/TJA_Signal1/81(NavSpdLimValue)
  RampDistance/1 -> HWA/ACC/TJA_Signal1/80(RampDistance)
  RoadCurvatureFar/1 -> HWA/ACC/TJA_Signal1/79(RoadCurvatureFar)
  TSR_Sign_Long_Distance/1 -> HWA/ACC/TJA_Signal1/78(TSR_Sign_Long_Distance)
  RoadCurvature/1 -> HWA/ACC/TJA_Signal1/77(dRoadCurvature)
  DrivingOnHighWay/1 -> HWA/ACC/TJA_Signal1/76(DrivingOnHighWay)
  HandsoffDetd/1 -> HWA/ACC/TJA_Signal1/75(HandsoffDetd)
  ACCTgtObjCntAlive/1 -> HWA/ACC/TJA_Signal1/74(ACCTgtObjCntAlive)
  Object_Orientation/1 -> HWA/ACC/TJA_Signal1/73(Object_Orientation)
  ObjMovingStateP0/1 -> HWA/ACC/TJA_Signal1/72(ObjMovingStateP0)
  ACCTgtObjAy/1 -> HWA/ACC/TJA_Signal1/71(ACCTgtObjAy)
  axAbsGroundP0/1 -> HWA/ACC/TJA_Signal1/70(axAbsGroundP0)
  vxRelP0/1 -> HWA/ACC/TJA_Signal1/69(vxRelP0)
  ACCTgtObjVy/1 -> HWA/ACC/TJA_Signal1/68(ACCTgtObjVy)
  ACCTgtObjExist/1 -> HWA/ACC/TJA_Signal1/67(ACCTgtObjExist)
  ACCTgtObjObstcl/1 -> HWA/ACC/TJA_Signal1/66(ACCTgtObjObstcl)
  ObjDYP0/1 -> HWA/ACC/TJA_Signal1/65(ObjDYP0)
  dxP0/1 -> HWA/ACC/TJA_Signal1/64(dxP0)
  IDP0/1 -> HWA/ACC/TJA_Signal1/63(IDP0)
  ACC_ParkShiftReq/1 -> HWA/ACC/TJA_Signal1/52(ACC_ParkShiftReq)
  ACC_DrvOffReq/1 -> HWA/ACC/TJA_Signal1/47(ACC_DrvOffReq)
  ISL_InterSysInfoDisp/1 -> HWA/ACC/TJA_Signal1/46(ISL_InterSysInfoDisp)
  ObjDYP3/1 -> HWA/ACC/TJA_Signal1/45(ObjDYP3)
  dxP3/1 -> HWA/ACC/TJA_Signal1/44(dxP3)
  ObjTypeP3/1 -> HWA/ACC/TJA_Signal1/43(ObjTypeP3)
  targetExistP3/1 -> HWA/ACC/TJA_Signal1/42(targetExistP3)
  ObjDYP2/1 -> HWA/ACC/TJA_Signal1/41(ObjDYP2)
  dxP2/1 -> HWA/ACC/TJA_Signal1/40(dxP2)
  ObjTypeP2/1 -> HWA/ACC/TJA_Signal1/39(ObjTypeP2)
  targetExistP2/1 -> HWA/ACC/TJA_Signal1/38(targetExistP2)
  ObjDYP1/1 -> HWA/ACC/TJA_Signal1/37(ObjDYP1)
  dxP1/1 -> HWA/ACC/TJA_Signal1/36(dxP1)
  ObjTypeP1/1 -> HWA/ACC/TJA_Signal1/35(ObjTypeP1)
  targetExistP1/1 -> HWA/ACC/TJA_Signal1/34(targetExistP1)
  ObjTypeP0/1 -> HWA/ACC/TJA_Signal1/33(ObjTypeP0)
  targetExistP0/1 -> HWA/ACC/TJA_Signal1/32(targetExistP0)
  ICA_HandsOffSwtResp/1 -> HWA/ACC/TJA_Signal1/31(ICA_HandsOffSwtResp)
  ACC_ISLResp/1 -> HWA/ACC/TJA_Signal1/30(ACC_ISLResp)
  HWA_LaneChangeReq/1 -> HWA/ACC/TJA_Signal1/28(HWA_LaneChangeReq)
  HWA_SnvtySet_Resp/1 -> HWA/ACC/TJA_Signal1/27(HWA_SnvtySet_Resp)
  DriverInloop_Monitor/1 -> HWA/ACC/TJA_Signal1/26(DriverInloop_Monitor)
  P1HeadingAngle/1 -> HWA/ACC/TJA_Signal1/25(P1HeadingAngle)
  fu_typeP1/1 -> HWA/ACC/TJA_Signal1/24(fu_typeP1)
  P3HeadingAngle/1 -> HWA/ACC/TJA_Signal1/23(P3HeadingAngle)
  fu_typeP3/1 -> HWA/ACC/TJA_Signal1/22(fu_typeP3)
  P2HeadingAngle/1 -> HWA/ACC/TJA_Signal1/21(P2HeadingAngle)
  fu_typeP2/1 -> HWA/ACC/TJA_Signal1/20(fu_typeP2)
  P0HeadingAngle/1 -> HWA/ACC/TJA_Signal1/19(P0HeadingAngle)
  fu_typeP0/1 -> HWA/ACC/TJA_Signal1/18(fu_typeP0)
  ACC_HazActv/1 -> HWA/ACC/TJA_Signal1/16(ACC_HazActv)
  TJA_ACC_SelSts/1 -> HWA/ACC/TJA_Signal1/14(TJA_ACC_SelSts)
  ACC_SpdSetValue/1 -> HWA/ACC/TJA_Signal1/13(ACC_SpdSetValue)
  ACC_TimeGapSet/1 -> HWA/ACC/TJA_Signal1/12(ACC_TimeGapSet)
  HWA_Warning/1 -> HWA/ACC/TJA_Signal1/11(HWAWarningLevel)
  HWA_Resp/1 -> HWA/ACC/TJA_Signal1/10(HWA_Resp)
  ALC_Resp/1 -> HWA/ACC/TJA_Signal1/9(ALC_Resp)
  TJATextDisp/1 -> HWA/ACC/TJA_Signal1/8(TJATextDisp)
  ACCTextDisp/1 -> HWA/ACC/TJA_Signal1/7(ACCTextDisp)
  HWA_ModeDisp/1 -> HWA/ACC/TJA_Signal1/6(HWA_ModeDisp)
  TJA_ModeDisp/1 -> HWA/ACC/TJA_Signal1/5(TJA_ModeDisp)
  ACC_ModeDisp/1 -> HWA/ACC/TJA_Signal1/4(ACC_ModeDisp)
  HWASts/1 -> HWA/ACC/TJA_Signal1/3(HWASts)
  TJASts/1 -> HWA/ACC/TJA_Signal1/2(TJASts)
  ACCSts/1 -> HWA/ACC/TJA_Signal1/1(ACCSts)
